simulink model "sinusoidal_pwm_three_phase_inverters"  (R2014b)
settings: Solver=ode23tb  StartTime=0.0  StopTime=0.3  MaxStep=1e-4  RelTol=1e-3
libraries: powerlib x13, powerlib_meascontrol x3
settings Model: SimulationMode=accelerator  Creator=Amr Saleh  LastModifiedBy=Amr Saleh

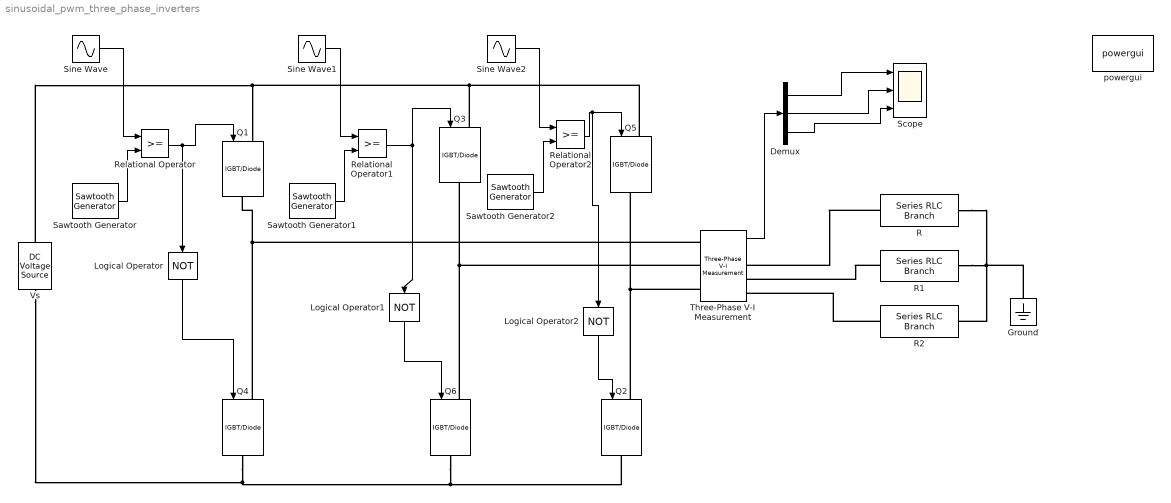
== system sinusoidal_pwm_three_phase_inverters ==
  Demux : Demux  Outputs=3
  Ground : powerlib/Elements/Ground  LConnTagsString=a
  Logical Operator : Logic  Operator=NOT  AllPortsSameDT=off  OutDataTypeStr=boolean
  Logical Operator1 : Logic  Operator=NOT  AllPortsSameDT=off  OutDataTypeStr=boolean
  Logical Operator2 : Logic  Operator=NOT  AllPortsSameDT=off  OutDataTypeStr=boolean
  Q{1..6} (6 alike) : powerlib/Power Electronics/IGBT//Diode  Ron=1e-3  Rs=1e5  Cs=inf  Measurements=off
  R : powerlib/Elements/Series RLC Branch  LConnTagsString=__new0  RConnTagsString=__new0  BranchType=R  Resistance=10  Inductance=1e-3  SetiL0=off  InitialCurrent=0  Capacitance=1e-6  Setx0=off  InitialVoltage=0  Measurements=None
  R1 : powerlib/Elements/Series RLC Branch  LConnTagsString=__new0  RConnTagsString=__new0  BranchType=R  Resistance=10  Inductance=1e-3  SetiL0=off  InitialCurrent=0  Capacitance=1e-6  Setx0=off  InitialVoltage=0  Measurements=None
  R2 : powerlib/Elements/Series RLC Branch  LConnTagsString=__new0  RConnTagsString=__new0  BranchType=R  Resistance=10  Inductance=1e-3  SetiL0=off  InitialCurrent=0  Capacitance=1e-6  Setx0=off  InitialVoltage=0  Measurements=None
  Relational Operator : RelationalOperator  OutDataTypeStr=boolean
  Relational Operator1 : RelationalOperator  OutDataTypeStr=boolean
  Relational Operator2 : RelationalOperator  OutDataTypeStr=boolean
  Sawtooth Generator : powerlib_meascontrol/Pulse & Signal Generators/Sawtooth Generator  Freq=1000  Phase=180  Ts=0
  Sawtooth Generator1 : powerlib_meascontrol/Pulse & Signal Generators/Sawtooth Generator  Freq=1000  Phase=180  Ts=0
  Sawtooth Generator2 : powerlib_meascontrol/Pulse & Signal Generators/Sawtooth Generator  Freq=1000  Phase=180  Ts=0
  Scope : Scope  NumInputPorts=3
      settings: YMin=-150~-5~-5  YMax=150~5~5
  Sine Wave : Sin  Amplitude=0.98  Frequency=2*pi*50  SampleTime=0
  Sine Wave1 : Sin  Amplitude=0.98  Frequency=2*pi*50  Phase=120*(pi/180)  SampleTime=0
  Sine Wave2 : Sin  Amplitude=0.98  Frequency=2*pi*50  Phase=240*(pi/180)  SampleTime=0
  Three-Phase V-I Measurement : powerlib/Measurements/Three-Phase V-I Measurement  VoltageMeasurement=phase-to-ground  SetLabelV=off  LabelV=Vabc  Vpu=off  VpuLL=off  CurrentMeasurement=yes  SetLabelI=off  LabelI=Iabc  Ipu=off  Pbase=100e6  Vbase=500e3  OutputType=Complex  PhasorSimulation=off  PSBequivalent=0
  Vs : powerlib/Electrical Sources/DC Voltage Source  Amplitude=100  Measurements=None
  powergui : powerlib/powergui  Priority=1  SimulationMode=Continuous  SolverType=Tustin/Backward Euler (TBE)  SampleTime=50e-6  frequency=60  SPID=off  DisableSnubberDevices=off  DisableRonSwitches=off  DisableVfSwitches=off  SwTol=0  DisplayEquations=off  Interpol=off  methode=off  Ts=100  frequencyindice=0  Pbase=100e6  ErrMax=1e-4  Iterations=50  UnitsV=kV  UnitsW=MW  FunctionMessages=off  echomessages=off  HookPort=off  EnableUseOfTLC=off  x0status=blocks  RestoreLinks=warning  ResistiveCurrentMeasurement=off  Frange=[0:2:500]  Ylog=off  Xlog=on  ShowGrid=off  save=off  variable=ZData  structure=Vo  ZoomFFT=off  StartTime=0.0  cycles=1  DisplayStyle=1  fundamental=50  FreqAxis=on  MaxFrequency=1000  frequencyindicesteady=1  RmsSteady=1  display=off
  wires:
  Three-Phase V-I Measurement/1 -> Demux/1
  Demux/1 -> Scope/1
  Demux/2 -> Scope/2
  Demux/3 -> Scope/3
  Sine Wave/1 -> Relational Operator/1
  Sawtooth Generator/1 -> Relational Operator/2
  Relational Operator/1 -> Q1/1, Logical Operator/1
  Sine Wave1/1 -> Relational Operator1/1
  Sawtooth Generator1/1 -> Relational Operator1/2
  Sine Wave2/1 -> Relational Operator2/1
  Sawtooth Generator2/1 -> Relational Operator2/2
  Relational Operator2/1 -> Q5/1, Logical Operator2/1
  Logical Operator/1 -> Q4/1
  Logical Operator1/1 -> Q6/1
  Relational Operator1/1 -> Q3/1, Logical Operator1/1
  Logical Operator2/1 -> Q2/1
  connections:
  Q5/LConn1 -- Vs/RConn1 -- Q1/LConn1 -- Q3/LConn1
  Q2/LConn1 -- Three-Phase V-I Measurement/LConn3 -- Q5/RConn1
  Q6/LConn1 -- Three-Phase V-I Measurement/LConn2 -- Q3/RConn1
  Q4/LConn1 -- Three-Phase V-I Measurement/LConn1 -- Q1/RConn1
  Q4/RConn1 -- Vs/LConn1 -- Q6/RConn1 -- Q2/RConn1
  R/RConn1 -- Ground/LConn1 -- R1/RConn1 -- R2/RConn1
  R/LConn1 -- Three-Phase V-I Measurement/RConn1
  R1/LConn1 -- Three-Phase V-I Measurement/RConn2
  R2/LConn1 -- Three-Phase V-I Measurement/RConn3
